simulink model "hw_bsc_rrtstar_pi"  (R2021b)
settings: Solver=ode1  StartTime=0.0  StopTime=100  FixedStep=0.01  RelTol=1e-3  EnableMultiTasking=on
undefined symbols (not defined in the file or in its folder): a, b, c, ki, kp, ux, uy
libraries: arduinolib x4, arduinosensorlib x2
settings Model: ExtModeTrigDuration=2  Creator=ONLY-GOD  LastModifiedBy=ASUS
settings SolverCC: AlgebraicLoopSolver=TrustRegion
settings OptimizationCC: EnhancedBackFolding=on  PassReuseOutputArgsAs=Individual arguments  ZeroExternalMemoryAtStartup=off  ZeroInternalMemoryAtStartup=off  MaxStackSize=64  OptimizeBlockOrder=speed  DifferentSizesBufferReuse=on  OptimizationCustomize=off  EfficientTunableParamExpr=on
settings DebuggingCC: ParameterTunabilityLossMsg=error  SFMachineParentedDataDiag=warning
settings HardwareCC: ProdBitPerPointer=32  ProdBitPerSizeT=32  ProdBitPerPtrDiffT=32  ProdLargestAtomicInteger=Long  ProdLargestAtomicFloat=Double  ProdWordSize=32  ProdHWDeviceType=ARM Compatible->ARM Cortex
settings SFSimCC: MATLABDynamicMemAlloc=off
settings RTWCC: Description=Embedded Coder  SystemTargetFile=ert.tlc  HardwareBoard=Arduino Due  TemplateMakefile=ert_default_tmf  Toolchain=Arduino ARM  BuildConfiguration=Faster Runs
settings CodeAppCC: ForceParamTrailComments=on  IgnoreCustomStorageClasses=off  OperatorAnnotations=on  SimulinkDataObjDesc=on  SFDataObjDesc=on  InsertBlockDesc=on
settings ERTTargetCC: SupportContinuousTime=on  SupportVariableSizeSignals=on  ExtModeTransport=3  ExtModeStaticAlloc=on  ExtModeStaticAllocSize=24576  ExtModeMexFile=ext_xcp  ExtModeIntrfLevel=Level2 - Open

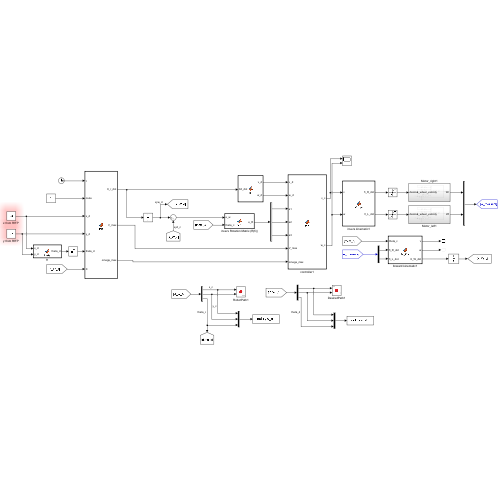
[thumbnail: Simulink's stored preview of the top-level diagram]
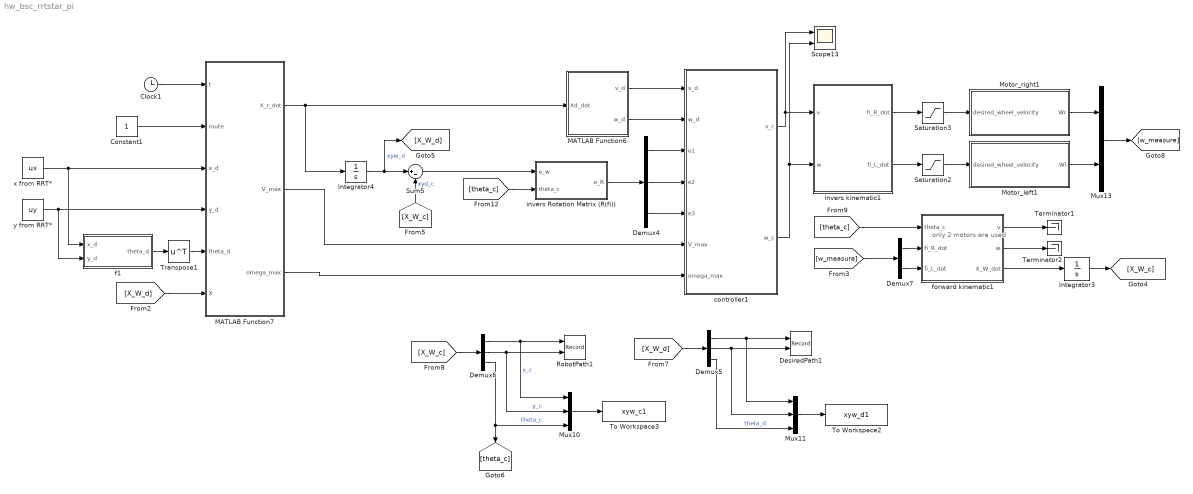
== system hw_bsc_rrtstar_pi ==
  note: only 2 motors are used
  Clock1 : Clock
  Constant1 : Constant
  Demux4 : Demux  Outputs=3
  Demux5 : Demux  Outputs=3
  Demux6 : Demux  Outputs=3
  Demux7 : Demux  Outputs=2
  DesiredPath1 : Record  FileSettingsInternal="{\"entries\":[{\"content\":{\"excelSettings\":{\"content\":{},\"type\":\"Streamout.ExcelSettings\"}},\"type\":\"Streamout.FileSettingStorage\",\"uuid\":\"d73c6bc3-906a-477a-a3ca-49659e58bbc0\"}],\"packageUris\":[\"http://schema.mathworks.com/mf0/streamout_blocks/R2020a\"],\"version\":\"1.0\"}"  Layout=[1 1]  SignalsInternal="{\"entries\":[{\"content\":{\"signals\":[{\"content\":{\"blockPath\":[\"hw_bsc_rrtstar_pi/DesiredPath1\"],\"channel\":[],\"dimensions\":[1],\"domain\":\"hw_bsc_rrtstar_pi/DesiredPath1\",\"lineColor\":\"#a2142f\",\"plots\":[],\"port\":1,\"sid\":[],\"signalID\":35,\"signalName\":\"Demux5:1\"},\"type\":\"RecordBlkView.Signal\",\"uuid\":\"7e275058-4173-4b43-af81-221a9d32ff05\"},{\"content\":{\"blockPath\":[\"hw_bsc_rrtstar_pi/DesiredPath1\"],\"channel\":[],\"dimensions\":[1],\"domain\":\"hw_bsc_rrtstar_pi/DesiredPath1\",\"lineColor\":\"#139fff\",\"plots\":[],\"port\":2,\"sid\":[],\"signalID\":38,\"signalName\":\"Demux5:2\"},\"type\":\"RecordBlkView.Signal\",\"uuid\":\"dc537f65-690b-48ac-9ebf-95fdd6f3a0ad\"}]},\"type\":\"RecordBlkView.InputSignals\",\"uuid\":\"b875a17a-627b-4dbc-878c-b398e2a06ca3\"}],\"packageUris\":[\"http://schema.mathworks.com/mf0/streamout_blocks/R2020a\"],\"version\":\"1.0\"}"  VisualizationBindings="{\"xyplotplugin\":{\"info\":[{\"series\":[],\"subplotID\":1}]}}"  CompatibilityTag=XY  st=-1
  Integrator3 : Integrator  InitialCondition=[0;0;0]
  Integrator4 : Integrator
  MATLAB Function6 : MATLAB Function  TreatAsAtomicUnit=on
  MATLAB Function7 : MATLAB Function  TreatAsAtomicUnit=on
  Motor_left1 : Subsystem
  Motor_right1 : Subsystem
  Mux10 : Mux  Inputs=3
  Mux11 : Mux  Inputs=3
  Mux13 : Mux  Inputs=2
  RobotPath1 : Record  FileSettingsInternal="{\"entries\":[{\"content\":{\"excelSettings\":{\"content\":{},\"type\":\"Streamout.ExcelSettings\"}},\"type\":\"Streamout.FileSettingStorage\",\"uuid\":\"64a05b15-e49c-4f92-bae4-adb1b6faa0e9\"}],\"packageUris\":[\"http://schema.mathworks.com/mf0/streamout_blocks/R2020a\"],\"version\":\"1.0\"}"  Layout=[1 1]  SignalsInternal="{\"entries\":[{\"content\":{\"signals\":[{\"content\":{\"blockPath\":[\"hw_bsc_rrtstar_pi/RobotPath1\"],\"channel\":[],\"dimensions\":[1],\"domain\":\"hw_bsc_rrtstar_pi/RobotPath1\",\"lineColor\":\"#a2142f\",\"plots\":[],\"port\":1,\"sid\":[],\"signalID\":27,\"signalName\":\"x_c\"},\"type\":\"RecordBlkView.Signal\",\"uuid\":\"57e800db-7c21-4fce-9f6f-754ff72fd0b2\"},{\"content\":{\"blockPath\":[\"hw_bsc_rrtstar_pi/RobotPath1\"],\"channel\":[],\"dimensions\":[1],\"domain\":\"hw_bsc_rrtstar_pi/RobotPath1\",\"lineColor\":\"#139fff\",\"plots\":[],\"port\":2,\"sid\":[],\"signalID\":30,\"signalName\":\"y_c\"},\"type\":\"RecordBlkView.Signal\",\"uuid\":\"39f88eed-cd09-4986-ba86-17572affd537\"}]},\"type\":\"RecordBlkView.InputSignals\",\"uuid\":\"672a287b-ff6f-43ae-b432-bcd62a67ece3\"}],\"packageUris\":[\"http://schema.mathworks.com/mf0/streamout_blocks/R2020a\"],\"version\":\"1.0\"}"  VisualizationBindings="{\"xyplotplugin\":{\"info\":[{\"series\":[],\"subplotID\":1}]}}"  CompatibilityTag=XY  st=-1
  Saturation2 : Saturate  UpperLimit=14  LowerLimit=-14
  Saturation3 : Saturate  UpperLimit=14  LowerLimit=-14
  Scope13 : Scope  NumInputPorts=2
  Sum5 : Sum  Inputs=|+-
  Terminator1 : Terminator
  Terminator2 : Terminator
  To Workspace2 : ToWorkspace  VariableName=xyw_d1  SaveFormat=Timeseries  SampleTime=-1
  To Workspace3 : ToWorkspace  VariableName=xyw_c1  SaveFormat=Timeseries  SampleTime=-1
  Transpose1 : Math  Operator=transpose  SaturateOnIntegerOverflow=on
  controller1 : MATLAB Function  TreatAsAtomicUnit=on
  f1 : MATLAB Function  TreatAsAtomicUnit=on
  forward kinematic1 : MATLAB Function  TreatAsAtomicUnit=on
  invers Rotation Matrix (R(fi)) : MATLAB Function  TreatAsAtomicUnit=on
  invers kinematic1 : MATLAB Function  TreatAsAtomicUnit=on
  x from RRT* : Constant  Value=ux
  y from RRT* : Constant  Value=uy
  wires:
  Demux4/1 -> controller1/3(e1)
  controller1/1(v_c) -> invers kinematic1/1(v), Scope13/1
  Constant1/1 -> MATLAB Function7/2(route)
  [X_W_d] -> MATLAB Function7/6(X)
  Demux5/1 -> Mux11/1, DesiredPath1/1
  forward kinematic1/1(v) -> Terminator1/1
  Transpose1/1 -> MATLAB Function7/5(theta_d)
  invers Rotation Matrix (R(fi))/1(e_R) -> Demux4/1
  forward kinematic1/3(X_W_dot) -> Integrator3/1
  [X_W_c] -> Sum5/2  "xyd_c"
  Mux11/1 -> To Workspace2/1
  Demux6/1 -> Mux10/1, RobotPath1/1  "x_c"
  Demux4/3 -> controller1/5(e3)
  Demux4/2 -> controller1/4(e2)
  Sum5/1 -> invers Rotation Matrix (R(fi))/1(e_w)
  Demux7/1 -> forward kinematic1/2(fi_R_dot)
  MATLAB Function7/1(X_r_dot) -> Integrator4/1, MATLAB Function6/1(Xd_dot)
  Demux6/3 -> Mux10/3, [theta_c]  "theta_c"
  [X_W_c] -> Demux6/1
  controller1/2(w_c) -> invers kinematic1/2(w), Scope13/2
  Integrator3/1 -> [X_W_c]
  Demux6/2 -> Mux10/2, RobotPath1/2  "y_c"
  forward kinematic1/2(w) -> Terminator2/1
  Demux7/2 -> forward kinematic1/3(fi_L_dot)
  Mux10/1 -> To Workspace3/1
  [w_measure] -> Demux7/1
  MATLAB Function6/1(v_d) -> controller1/1(v_d)
  [theta_c] -> forward kinematic1/1(theta_c)
  [X_W_d] -> Demux5/1
  MATLAB Function6/2(w_d) -> controller1/2(w_d)
  Demux5/3 -> Mux11/3  "theta_d"
  f1/1(theta_d) -> Transpose1/1
  Clock1/1 -> MATLAB Function7/1(t)
  Integrator4/1 -> [X_W_d], Sum5/1  "xyw_d"
  Demux5/2 -> Mux11/2, DesiredPath1/2
  [theta_c] -> invers Rotation Matrix (R(fi))/2(theta_c)
  invers kinematic1/1(fi_R_dot) -> Saturation3/1
  invers kinematic1/2(fi_L_dot) -> Saturation2/1
  Saturation3/1 -> Motor_right1/1(desired_wheel_velocity)
  Saturation2/1 -> Motor_left1/1(desired_wheel_velocity)
  Motor_right1/1(Wr) -> Mux13/1
  Motor_left1/1(Wl) -> Mux13/2
  Mux13/1 -> [w_measure]
  x from RRT*/1 -> f1/1(x_d), MATLAB Function7/3(x_d)
  y from RRT*/1 -> f1/2(y_d), MATLAB Function7/4(y_d)
  MATLAB Function7/2(V_max) -> controller1/6(V_max)
  MATLAB Function7/3(omega_max) -> controller1/7(omega_max)

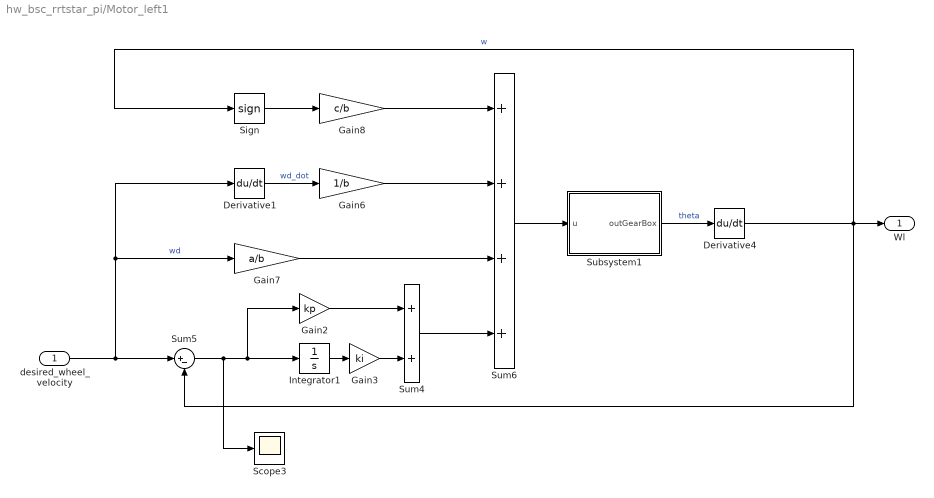
== system hw_bsc_rrtstar_pi/Motor_left1 ==
  desired_wheel_velocity : Inport
  Derivative1 : Derivative
  Derivative4 : Derivative
  Gain2 : Gain  Gain=kp
  Gain3 : Gain  Gain=ki
  Gain6 : Gain  Gain=1/b
  Gain7 : Gain  Gain=a/b
  Gain8 : Gain  Gain=c/b
  Integrator1 : Integrator
  Scope3 : Scope
  Sign : Signum
  Subsystem1 : Subsystem
  Sum4 : Sum
  Sum5 : Sum  Inputs=|+-
  Sum6 : Sum  Inputs=++++
  Wl : Outport
  wires:
  Gain8/1 -> Sum6/1
  Gain6/1 -> Sum6/2
  Sum5/1 -> Gain2/1, Integrator1/1, Scope3/1
  Gain2/1 -> Sum4/1
  Derivative1/1 -> Gain6/1  "wd_dot"
  Gain7/1 -> Sum6/3
  Gain3/1 -> Sum4/2
  Sign/1 -> Gain8/1
  Derivative4/1 -> Wl/1, Sign/1, Sum5/2  "w"
  desired_wheel_velocity/1 -> Sum5/1, Gain7/1, Derivative1/1  "wd"
  Subsystem1/1(outGearBox) -> Derivative4/1  "theta"
  Integrator1/1 -> Gain3/1
  Sum4/1 -> Sum6/4
  Sum6/1 -> Subsystem1/1(u)

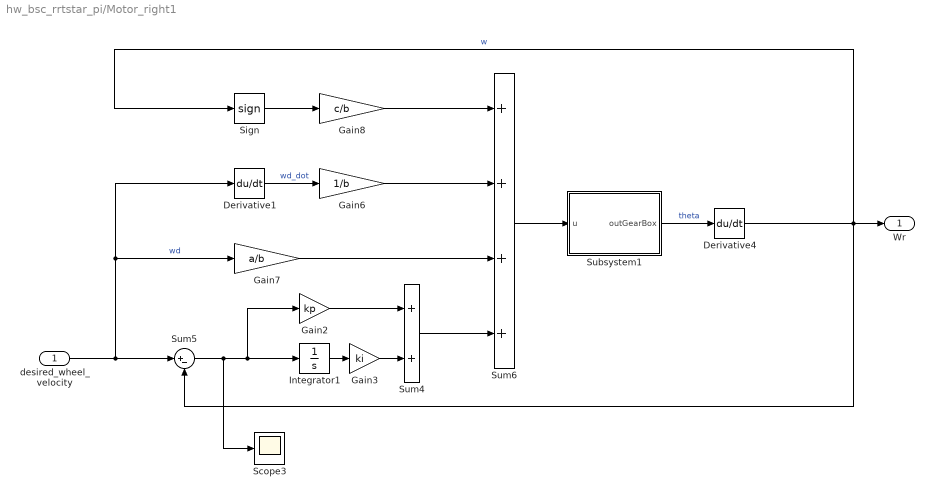
== system hw_bsc_rrtstar_pi/Motor_right1 ==
  desired_wheel_velocity : Inport
  Derivative1 : Derivative
  Derivative4 : Derivative
  Gain2 : Gain  Gain=kp
  Gain3 : Gain  Gain=ki
  Gain6 : Gain  Gain=1/b
  Gain7 : Gain  Gain=a/b
  Gain8 : Gain  Gain=c/b
  Integrator1 : Integrator
  Scope3 : Scope
  Sign : Signum
  Subsystem1 : Subsystem
  Sum4 : Sum
  Sum5 : Sum  Inputs=|+-
  Sum6 : Sum  Inputs=++++
  Wr : Outport
  wires:
  Gain8/1 -> Sum6/1
  Gain6/1 -> Sum6/2
  Sum5/1 -> Gain2/1, Integrator1/1, Scope3/1
  Gain2/1 -> Sum4/1
  Derivative1/1 -> Gain6/1  "wd_dot"
  Gain7/1 -> Sum6/3
  Gain3/1 -> Sum4/2
  Sign/1 -> Gain8/1
  Derivative4/1 -> Wr/1, Sign/1, Sum5/2  "w"
  desired_wheel_velocity/1 -> Sum5/1, Gain7/1, Derivative1/1  "wd"
  Subsystem1/1(outGearBox) -> Derivative4/1  "theta"
  Integrator1/1 -> Gain3/1
  Sum4/1 -> Sum6/4
  Sum6/1 -> Subsystem1/1(u)

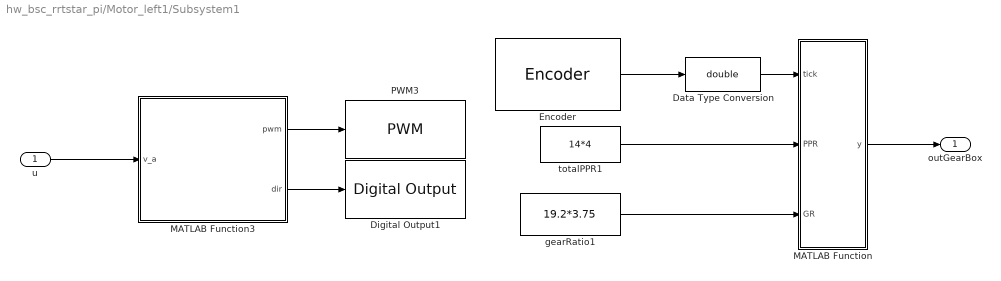
== system hw_bsc_rrtstar_pi/Motor_left1/Subsystem1 ==
  u : Inport
  Data Type Conversion : DataTypeConversion  OutDataTypeStr=double
  Digital Output1 : arduinolib/Digital Output  pinNumber=4  Direction=output  blockPlatform=arduino
  Encoder : arduinosensorlib/Encoder  InputA=10  InputB=11  Mode=No reset  SampleTime=-1
      settings: SourceProductBaseCode=ARDUINO
  MATLAB Function : MATLAB Function  TreatAsAtomicUnit=on
  MATLAB Function3 : MATLAB Function  TreatAsAtomicUnit=on
  PWM3 : arduinolib/PWM  pinNumber=5  frequencyType=Default  desiredFrequency=490.2  achievableFrequency=490.2
  gearRatio1 : Constant  Value=19.2*3.75
  totalPPR1 : Constant  Value=14*4
  outGearBox : Outport
  wires:
  MATLAB Function3/1(pwm) -> PWM3/1
  u/1 -> MATLAB Function3/1(v_a)
  MATLAB Function/1(y) -> outGearBox/1
  MATLAB Function3/2(dir) -> Digital Output1/1
  totalPPR1/1 -> MATLAB Function/2(PPR)
  Data Type Conversion/1 -> MATLAB Function/1(tick)
  gearRatio1/1 -> MATLAB Function/3(GR)
  Encoder/1 -> Data Type Conversion/1

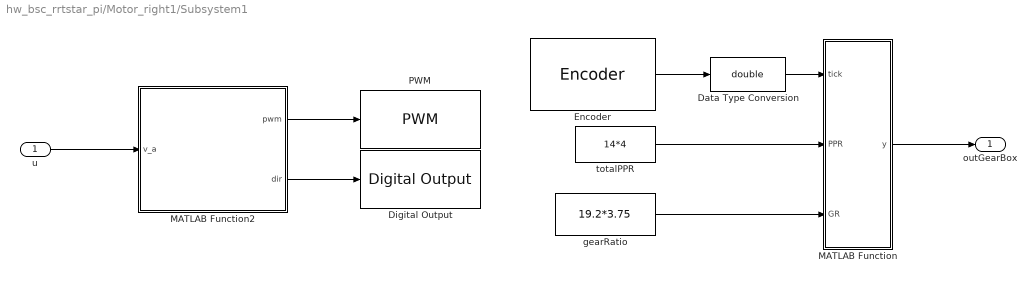
== system hw_bsc_rrtstar_pi/Motor_right1/Subsystem1 ==
  u : Inport
  Data Type Conversion : DataTypeConversion  OutDataTypeStr=double
  Digital Output : arduinolib/Digital Output  pinNumber=7  Direction=output  blockPlatform=arduino
  Encoder : arduinosensorlib/Encoder  InputA=8  InputB=9  Mode=No reset  SampleTime=-1
      settings: SourceProductBaseCode=ARDUINO
  MATLAB Function : MATLAB Function  TreatAsAtomicUnit=on
  MATLAB Function2 : MATLAB Function  TreatAsAtomicUnit=on
  PWM : arduinolib/PWM  pinNumber=6  frequencyType=Default  desiredFrequency=490.2  achievableFrequency=490.2
  gearRatio : Constant  Value=19.2*3.75
  totalPPR : Constant  Value=14*4
  outGearBox : Outport
  wires:
  MATLAB Function/1(y) -> outGearBox/1
  MATLAB Function2/2(dir) -> Digital Output/1
  Encoder/1 -> Data Type Conversion/1
  u/1 -> MATLAB Function2/1(v_a)
  gearRatio/1 -> MATLAB Function/3(GR)
  totalPPR/1 -> MATLAB Function/2(PPR)
  MATLAB Function2/1(pwm) -> PWM/1
  Data Type Conversion/1 -> MATLAB Function/1(tick)

== matlab function hw_bsc_rrtstar_pi/f1 ==
  data: theta_d output; x_d input; y_d input
function theta_d = theta( x_d, y_d)
theta_d = zeros(1,length(x_d));
for i = 1:length(x_d)-1
       theta_d(i) = atan2(y_d (i+1) - y_d(i), x_d(i+1) - x_d(i));
end

== matlab function hw_bsc_rrtstar_pi/forward kinematic1 ==
  data: v output; w output; theta_c input; fi_R_dot input; X_W_dot output; fi_L_dot input
function [v, w, X_W_dot] = M_inv(theta_c,fi_R_dot, fi_L_dot)
r = 0.07;      %wheel radius
b = 0.22; 

w = r*[0.5/b -0.5/b]*[fi_R_dot; fi_L_dot];
v = r*[0.5 0.5]*[fi_R_dot; fi_L_dot];
X_W_dot = [cos(theta_c) 0;sin(theta_c) 0; 0 1]*[v; w];

== matlab function hw_bsc_rrtstar_pi/invers Rotation Matrix (R(fi)) ==
  data: e_w input; theta_c input; e_R output
function e_R = fcn(e_w,theta_c)
%#codegen

R = [cos(theta_c), sin(theta_c), 0; -sin(theta_c), cos(theta_c), 0; 0, 0, 1];
e_R = R*e_w;

== matlab function hw_bsc_rrtstar_pi/invers kinematic1 ==
  data: v input; fi_R_dot output; w input; fi_L_dot output
function [fi_R_dot, fi_L_dot] = M_inv(v, w)
r = 0.07;      %wheel radius
b = 0.22; 
fi_R_dot = (v + w*b)/r;
fi_L_dot = (v - w*b)/r;

== matlab function hw_bsc_rrtstar_pi/Motor_left1/Subsystem1/MATLAB Function ==
  data: tick input; y output; PPR input; GR input
function y = fcn(tick,PPR,GR)

y = (2*pi*tick)/(PPR*GR);

== matlab function hw_bsc_rrtstar_pi/Motor_right1/Subsystem1/MATLAB Function ==
  data: tick input; y output; PPR input; GR input
function y = fcn(tick,PPR,GR)

y = (2*pi*tick)/(PPR*GR);

== matlab function hw_bsc_rrtstar_pi/Motor_right1/Subsystem1/MATLAB Function2 ==
  data: v_a input; pwm output; dir output
function [pwm,dir] = fcn(v_a)

vmax = 22.9;
pwm_cal = v_a*254/vmax;
if pwm_cal > 0
    pwm = pwm_cal;
    dir = 0;
elseif pwm_cal < 0
    pwm = abs(pwm_cal);
    dir = 1;
else
    pwm = 0;
    dir = 0;
end

== matlab function hw_bsc_rrtstar_pi/Motor_left1/Subsystem1/MATLAB Function3 ==
  data: v_a input; pwm output; dir output
function [pwm,dir] = fcn(v_a)

vmax = 22.9;
pwm_cal = v_a*254/vmax;
if pwm_cal > 0
    pwm = pwm_cal;
    dir = 1;
elseif pwm_cal < 0
    pwm = abs(pwm_cal);
    dir = 0;
else
    pwm = 0;
    dir = 0;
end

== matlab function hw_bsc_rrtstar_pi/MATLAB Function6 ==
  data: Xd_dot input; v_d output; w_d output
function [v_d, w_d] = fcn(Xd_dot)

v_d = sqrt(Xd_dot(1)^2 + Xd_dot(2)^2);
w_d = Xd_dot(3);

== matlab function hw_bsc_rrtstar_pi/MATLAB Function7 ==
  settings: updateMethod=DISCRETE
  data: t input; route input; x_d input; y_d input; theta_d input; X_r_dot output; X input; V_max output; omega_max output
function [X_r_dot, V_max, omega_max]   = fcn(t,route,x_d,y_d,theta_d, X)
%#codegen

persistent k i j X_p_i omega_p_j t1 t2
if isempty(k)
    i = int8(1);
    j = int8(1);
    X_p_i = [0;0];
    omega_p_j = 0;
    t1 = t;
    t2 = t;
    k = 1;
end
tau = 0.15;
tau1 = 0.15;
V_max = 0.6; % maximum velocity0.2
a = 5;      % acceleration0.1
omega_max = 2; %0.15
alpha = 1; %0.1

X_r_dot = zeros(3,1);
switch route
    case 1
%         X_p = [1.5   1.5  0];
%%%%%%%%%%%%%theta_d = zeros(length(x),1);
        X_p = [x_d,y_d,theta_d]; % X_p = [x,y,theta];
    otherwise
        X_r_dot = [0;0;0];
        return;
end
X_p = X_p'; % X_p = [x;y;theta]
[~,col] = size(X_p);
dX = X_p(1:2,i)-X_p_i;
norm_dX = norm(dX);
two_rmin = V_max^2/a;  
dtheta = X_p(3,j)-omega_p_j;
norm_dtheta = abs(dtheta);
two_thetamin = omega_max^2/alpha; 

if norm_dX > two_rmin
    ta = V_max/a;                   % acceleration period
    tad = (norm_dX-two_rmin)/V_max; % acc to deceleration period
    td = ta + tad;                  % start deceleration
    te = ta + td;                   % end deceleration
    if (t-t1) < ta
        v = a*(t-t1);
    elseif ta <= (t-t1) && (t-t1) < td
        v = V_max;
    elseif td <= (t-t1) && (t-t1) < te
        v = -a*(t-t1-td) + V_max;
    else
        v = 0;
    end
else
    tp = sqrt(norm_dX/a);
    te = 2*tp;
    Vp = a*tp;
    if (t-t1) < tp
        v = a*(t-t1);
    elseif tp < (t-t1) && (t-t1) < te
        v = -a*(t-t1-tp)+Vp;
    else
        v = 0;
    end
end
if norm_dX~=0
    X_r_dot(1:2) = v*dX/norm_dX;
end

dist_X = norm(X_p(1:2,i)-X(1:2));
if (i<col)&&(dist_X < tau)
    X_p_i = X(1:2);
    t1    = t;
    i     = i+1;
end

if norm_dtheta > two_thetamin
    ta = omega_max/alpha;                   % acceleration period
    tad = (norm_dtheta-two_thetamin)/omega_max; % acc to deceleration period
    td = ta + tad;                  % start deceleration
    te = ta + td;                   % end deceleration
    if (t-t2) < ta
        omega = alpha*(t-t2);
    elseif ta <= (t-t2) && (t-t2) < td
        omega = omega_max;
    elseif td <= (t-t2) && (t-t2) < te
        omega = -alpha*(t-t2-td) + omega_max;
    else
        omega = 0;
    end
else
    tp = sqrt(norm_dtheta/alpha);
    te = 2*tp;
    omegap = alpha*tp;
    if (t-t2) < tp
        omega = alpha*(t-t2);
    elseif tp < (t-t2) && (t-t2) < te
        omega = -alpha*(t-t2-tp)+omegap;
    else
        omega = 0;
    end
end
X_r_dot(3) = omega*sign(dtheta);

dist_theta = abs(X_p(3,j)-X(3));
if (j<col)&&(dist_theta < tau1)
    omega_p_j = X(3);
    t2    = t;
    j     = j+1;
end

== matlab function hw_bsc_rrtstar_pi/controller1 ==
  data: v_d input; w_d input; e1 input; e2 input; e3 input; v_c output; w_c output; V_max input; omega_max input
function [v_c,w_c] =  fcn(v_d, w_d, e1, e2, e3, V_max, omega_max)            

k1 = 4; %1
k2 = 30; %20
k3 = 6; %1
%lambda = 2 ;

% x_e_hat = e1 - k1*w*e2;
% v1 = w*e2 + v_d*cos(e3) - v - k1*w_dot*e2 + k1*w*(w*e1 - v_d*sin(e3));
% v_c = v1 - e2*w + k2*x_e_hat;
% w_c = w_d + lambda*e2*v_d*i + k3*lambda*e3;
%w_c = w_d +k3*lambda*e3;

v_c = k1*e1 + v_d*cos(e3);
w_c = w_d + k2*v_d*e2 + k3*v_d*sin(e3);

if v_c > V_max, v_c = V_max; end
if w_c > omega_max, w_c = omega_max; end
